simulink model "gm_sampleModel1831_sub"  (R2023a)
settings: Solver=VariableStepAuto  StartTime=0.0  StopTime=10.0  RelTol=1e-3
libraries: simulink x1
settings Model: Creator=user1  LastModifiedBy=user1
settings OptimizationCC: BlockReduction=off  ConditionallyExecuteInputs=off
settings DebuggingCC: InheritedTsInSrcMsg=none

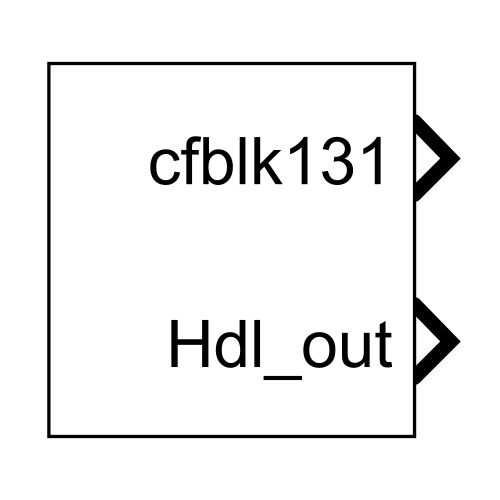
[thumbnail: Simulink's stored preview of the top-level diagram]
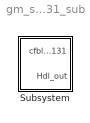
== system gm_sampleModel1831_sub ==
  Subsystem : Subsystem

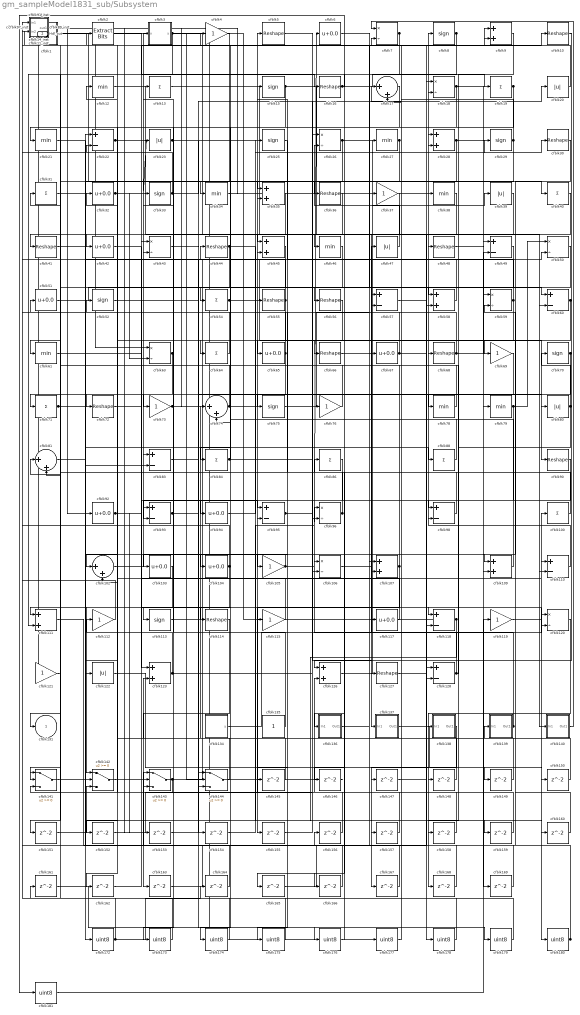
== system gm_sampleModel1831_sub/Subsystem ==
  cfblk1 : Subsystem  mask(Detect Rise Nonnegative){vinit=double(0), InputProcessing=Elements as channels (sample based), OutDataTypeStr=uint8}
      mask prompts: vinit "Simulink:masks:InitialCondition_MP"; InputProcessing "Simulink:masks:InputProcessing_MP"; OutDataTypeStr "Simulink:masks:OutputDataType_MP"
      mask help: Simulink:masks:DetectRiseNonnegative_MD
      mask init:
      | InputProcessing = 'Elements as channels (sample based)';
      | OutDataTypeStr = 'uint8';
      | vinit = double(0);
      mask TypeOptions InputProcessing: Simulink:masks:ColumnsAsChannelsFrameBased | Simulink:masks:ElementsAsChannelsSampleBased
      mask TypeOptions OutDataTypeStr: Simulink:masks:uint8 | Simulink:masks:boolean
      mask Display: fprintf('U >= 0\n&  NOT\nU/z >= 0')
  cfblk{5,10,16,30,36,41,44,48,55..56,66,68,72,90,114,127} (16 alike) : Reshape
  cfblk{13,19,31,40,54,64,71,84,86,88,100} (11 alike) : Sum  Inputs=+  OutDataTypeStr=uint8
  cfblk{17,74,81,102} (4 alike) : Sum  Inputs=|++  OutDataTypeStr=uint8
  cfblk{6,32,42,51,65,67,92,94,103..104,117} (11 alike) : Bias  Bias=0.0  SaturateOnIntegerOverflow=off
  cfblk{4,37,69,73,76,105,112,115,119,121} (10 alike) : Gain  OutDataTypeStr=uint8
  cfblk{7,18,26,43,50,59,63,96,106,120} (10 alike) : Product  Inputs=*/  OutDataTypeStr=uint8  RndMeth=Zero  SaturateOnIntegerOverflow=on
  cfblk{9,28,35,45,58,107,109,111,123,126} (10 alike) : Sum  OutDataTypeStr=uint8
  cfblk108_inst : Subsystem
  cfblk{22,49,57,60,83,93,95,98,110,118,128} (11 alike) : Sum  Inputs=+-  OutDataTypeStr=uint8
  cfblk{8,15,25,29,33,52,70,75,113} (9 alike) : Signum
  cfblk116_inst : Subsystem
  cfblk11_inst : Subsystem
  cfblk{12,21,27,34,38,46,61,78..79} (9 alike) : MinMax  OutDataTypeStr=uint8
  cfblk{20,23,39,47,80,122} (6 alike) : Abs  OutDataTypeStr=uint8  SaturateOnIntegerOverflow=off
  cfblk134 : Subsystem  mask(Counter Free-Running){NumBits=double(16), tsamp=double(-1)}
      mask prompts: NumBits "Simulink:masks:NumberOfBits_MP"; tsamp "Simulink:masks:SampleTime_MP"
      mask help: Simulink:masks:CounterFreeRunning_MD
  cfblk135 : Constant  OutDataTypeStr=uint8  SampleTime=-1
  cfblk136 : Subsystem
  cfblk137 : Subsystem
  cfblk138 : Subsystem
  cfblk139 : Subsystem
  cfblk140 : Subsystem
  cfblk{141..144} (4 alike) : Switch  OutDataTypeStr=uint8  SaturateOnIntegerOverflow=off  InputSameDT=off
  cfblk{145..169} (25 alike) : Delay  SampleTime=1
  cfblk14_inst : Subsystem
  cfblk{172..181} (10 alike) : DataTypeConversion  OutDataTypeStr=uint8  SaturateOnIntegerOverflow=off  RndMeth=Floor
  cfblk2 : simulink/Logic and Bit Operations/Extract Bits  bitsToExtract=Upper half  numBits=8  bitIdxRange=[0 7]  outScalingMode=Preserve fixed-point scaling
      settings: LibrarySourceBlock=|
      | hdlsllib/Logic and Bit
      | Operations/Extract Bits
  cfblk3 : Subsystem  mask(Compare To Zero){relop=<=, OutDataTypeStr=uint8, ZeroCross=on}
      mask prompts: relop "Simulink:masks:Operator_MP"; OutDataTypeStr "Simulink:masks:OutputDataType_MP"; ZeroCross "Simulink:masks:EnableZerocrossingDetection_MP"
      mask help: Simulink:masks:CompareToZero_MD
      mask init:
      | OutDataTypeStr = 'uint8';
      | ZeroCross = 'on';
      | blkName = 'sampleModel1831_sub/Subsystem/cfblk3';
      | relop = '<=';
      | setValue = 'fixdt(0, 8)';
      mask TypeOptions relop: == | ~= | < | <= | >= | >
      mask TypeOptions OutDataTypeStr: Simulink:masks:uint8 | Simulink:masks:boolean
      mask Callback ZeroCross: sl('zeroCrossEnable', gcbh);
      mask Display: disp([relop,' 0'])
  cfblk89_inst : Subsystem
  cfblk91_inst : Subsystem
  cfblk97_inst : Subsystem
  cfblk131 : Outport  OutDataTypeStr=uint8  SampleTime=1  VectorParamsAs1DForOutWhenUnconnected=off
  Hdl_out : Outport  Port=2  OutDataTypeStr=uint8  SampleTime=1
  wires:
  cfblk1/1(Y) -> cfblk40/1
  cfblk10/1 -> cfblk126/1
  cfblk100/1 -> cfblk108_inst/2(in2)
  cfblk102/1 -> cfblk3/1(u)
  cfblk103/1 -> cfblk142/1
  cfblk104/1 -> cfblk97_inst/2(in2), cfblk111/1
  cfblk105/1 -> cfblk6/1, cfblk103/1
  cfblk106/1 -> cfblk39/1
  cfblk107/1 -> cfblk43/2, cfblk155/1
  cfblk108_inst/1(out1) -> cfblk121/1
  cfblk109/1 -> cfblk44/1
  cfblk11_inst/1(out1) -> cfblk154/1
  cfblk110/1 -> cfblk8/1
  cfblk111/1 -> cfblk156/1
  cfblk112/1 -> cfblk116_inst/2(in2)
  cfblk113/1 -> cfblk118/1
  cfblk114/1 -> cfblk163/1
  cfblk115/1 -> cfblk116_inst/1(in1)
  cfblk116_inst/1(out1) -> cfblk63/1
  cfblk117/1 -> cfblk32/1
  cfblk118/1 -> cfblk165/1, Hdl_out/1
  cfblk119/1 -> cfblk180/1
  cfblk12/1 -> cfblk137/1(In1)
  cfblk120/1 -> cfblk168/1
  cfblk121/1 -> cfblk31/1
  cfblk122/1 -> cfblk148/1
  cfblk123/1 -> cfblk28/1, cfblk112/1
  cfblk126/1 -> cfblk29/1
  cfblk127/1 -> cfblk18/1
  cfblk128/1 -> cfblk68/1, cfblk47/1
  cfblk13/1 -> cfblk46/1
  cfblk134/1(y) -> cfblk100/1
  cfblk135/1 -> cfblk83/1
  cfblk136/1(Out1) -> cfblk67/1
  cfblk137/1(Out1) -> cfblk149/1
  cfblk138/1(Out1) -> cfblk167/1
  cfblk139/1(Out1) -> cfblk98/2, cfblk106/1
  cfblk14_inst/1(out1) -> cfblk92/1
  cfblk140/1(Out1) -> cfblk7/1
  cfblk141/1 -> cfblk50/2
  cfblk142/1 -> cfblk143/1
  cfblk143/1 -> cfblk5/1, cfblk141/3
  cfblk144/1 -> cfblk123/2
  cfblk145/1 -> cfblk22/2
  cfblk146/1 -> cfblk1/1(U)
  cfblk147/1 -> cfblk9/1
  cfblk148/1 -> cfblk35/2
  cfblk149/1 -> cfblk7/2
  cfblk15/1 -> cfblk140/1(In1), cfblk54/1
  cfblk150/1 -> cfblk74/1
  cfblk151/1 -> cfblk142/3
  cfblk152/1 -> cfblk26/1
  cfblk153/1 -> cfblk45/2
  cfblk154/1 -> cfblk96/1
  cfblk155/1 -> cfblk110/1
  cfblk156/1 -> cfblk143/2
  cfblk157/1 -> cfblk126/2
  cfblk158/1 -> cfblk102/2
  cfblk159/1 -> cfblk95/2
  cfblk16/1 -> cfblk181/1, cfblk19/1
  cfblk160/1 -> cfblk59/2
  cfblk161/1 -> cfblk179/1
  cfblk162/1 -> cfblk107/2
  cfblk163/1 -> cfblk58/2
  cfblk164/1 -> cfblk43/1
  cfblk165/1 -> cfblk128/2
  cfblk166/1 -> cfblk143/3
  cfblk167/1 -> cfblk142/2
  cfblk168/1 -> cfblk57/1
  cfblk169/1 -> cfblk91_inst/2(in2)
  cfblk17/1 -> cfblk162/1
  cfblk172/1 -> cfblk108_inst/1(in1), cfblk164/1
  cfblk173/1 -> cfblk81/1
  cfblk174/1 -> cfblk81/2
  cfblk175/1 -> cfblk161/1
  cfblk176/1 -> cfblk86/1
  cfblk177/1 -> cfblk57/2
  cfblk178/1 -> cfblk89_inst/1(in1)
  cfblk179/1 -> cfblk89_inst/2(in2)
  cfblk18/1 -> cfblk49/1, cfblk158/1, cfblk21/1
  cfblk180/1 -> cfblk107/1, cfblk139/1(In1)
  cfblk181/1 -> cfblk119/1
  cfblk19/1 -> cfblk42/1, cfblk173/1
  cfblk2/1 -> cfblk16/1
  cfblk20/1 -> cfblk2/1
  cfblk21/1 -> cfblk157/1
  cfblk22/1 -> cfblk35/1, cfblk169/1
  cfblk23/1 -> cfblk144/1, cfblk59/1
  cfblk25/1 -> cfblk65/1
  cfblk26/1 -> cfblk28/2, cfblk84/1
  cfblk27/1 -> cfblk93/2, cfblk45/1
  cfblk28/1 -> cfblk151/1, cfblk150/1
  cfblk29/1 -> cfblk97_inst/1(in1), cfblk61/1
  cfblk3/1(y) -> cfblk178/1, cfblk141/2
  cfblk30/1 -> cfblk109/1
  cfblk31/1 -> cfblk34/1
  cfblk32/1 -> cfblk23/1, cfblk63/2, cfblk106/2
  cfblk33/1 -> cfblk14_inst/1(in1), cfblk18/2
  cfblk34/1 -> cfblk25/1
  cfblk35/1 -> cfblk72/1
  cfblk36/1 -> cfblk96/2
  cfblk37/1 -> cfblk146/1
  cfblk38/1 -> cfblk41/1
  cfblk39/1 -> cfblk98/1
  cfblk4/1 -> cfblk73/1
  cfblk40/1 -> cfblk105/1
  cfblk41/1 -> cfblk83/2
  cfblk42/1 -> cfblk118/2
  cfblk43/1 -> cfblk78/1
  cfblk44/1 -> cfblk144/3, cfblk160/1, cfblk159/1
  cfblk45/1 -> cfblk74/2
  cfblk46/1 -> cfblk94/1
  cfblk47/1 -> cfblk26/2
  cfblk48/1 -> cfblk79/1
  cfblk49/1 -> cfblk71/1
  cfblk5/1 -> cfblk69/1
  cfblk50/1 -> cfblk131/1
  cfblk51/1 -> cfblk60/1
  cfblk52/1 -> cfblk117/1
  cfblk54/1 -> cfblk90/1, cfblk37/1
  cfblk55/1 -> cfblk14_inst/2(in2), cfblk64/1
  cfblk56/1 -> cfblk102/1
  cfblk57/1 -> cfblk128/1
  cfblk58/1 -> cfblk15/1
  cfblk59/1 -> cfblk48/1, cfblk144/2
  cfblk6/1 -> cfblk60/2
  cfblk60/1 -> cfblk174/1, cfblk104/1
  cfblk61/1 -> cfblk95/1
  cfblk63/1 -> cfblk141/1, cfblk152/1
  cfblk64/1 -> cfblk12/1
  cfblk65/1 -> cfblk52/1, cfblk114/1
  cfblk66/1 -> cfblk10/1
  cfblk67/1 -> cfblk91_inst/1(in1), cfblk120/2
  cfblk68/1 -> cfblk49/2, cfblk17/1
  cfblk69/1 -> cfblk136/1(In1)
  cfblk7/1 -> cfblk56/1, cfblk111/2
  cfblk70/1 -> cfblk122/1, cfblk110/2
  cfblk71/1 -> cfblk109/2, cfblk88/1
  cfblk72/1 -> cfblk9/2
  cfblk73/1 -> cfblk75/1, cfblk113/1
  cfblk74/1 -> cfblk80/1, cfblk147/1, cfblk13/1
  cfblk75/1 -> cfblk27/1
  cfblk76/1 -> cfblk22/1
  cfblk78/1 -> cfblk51/1
  cfblk79/1 -> cfblk93/1, cfblk50/1
  cfblk8/1 -> cfblk66/1, cfblk36/1, cfblk166/1
  cfblk80/1 -> cfblk70/1, cfblk138/1(In1)
  cfblk81/1 -> cfblk172/1
  cfblk83/1 -> cfblk115/1
  cfblk84/1 -> cfblk4/1, cfblk120/1
  cfblk86/1 -> cfblk175/1
  cfblk88/1 -> cfblk11_inst/1(in1)
  cfblk89_inst/1(out1) -> cfblk177/1
  cfblk9/1 -> cfblk58/1
  cfblk90/1 -> cfblk145/1
  cfblk91_inst/1(out1) -> cfblk76/1
  cfblk92/1 -> cfblk123/1, cfblk153/1
  cfblk93/1 -> cfblk33/1, cfblk176/1
  cfblk94/1 -> cfblk30/1
  cfblk95/1 -> cfblk20/1, cfblk127/1
  cfblk96/1 -> cfblk55/1, cfblk11_inst/2(in2)
  cfblk97_inst/1(out1) -> cfblk38/1
  cfblk98/1 -> cfblk17/2

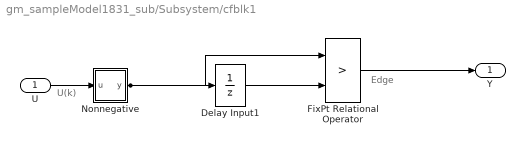
== system gm_sampleModel1831_sub/Subsystem/cfblk1 ==
  note: U(k)
  note: Edge
  U : Inport  OutDataTypeStr=uint8  SampleTime=1
  Delay Input1 : UnitDelay  Description=Store in Global RAM  DisableCoverage=on  InitialCondition=vinit  SampleTime=-1  HasFrameUpgradeWarning=on
  FixPt Relational Operator : RelationalOperator  Operator=>  OutDataTypeStr=fixdt(0, 8)  ZeroCross=off  InputSameDT=off
  Nonnegative : Subsystem  mask(Compare To Zero){relop=>=, OutDataTypeStr=boolean, ZeroCross=off}
      mask prompts: relop "Simulink:masks:Operator_MP"; OutDataTypeStr "Simulink:masks:OutputDataType_MP"; ZeroCross "Simulink:masks:EnableZerocrossingDetection_MP"
      mask help: Simulink:masks:CompareToZero_MD
      mask init:
      | OutDataTypeStr = 'boolean';
      | ZeroCross = 'off';
      | blkName = 'sampleModel1831_sub/Subsystem/cfblk1/Nonnegative';
      | relop = '>=';
      | setValue = 'boolean';
      mask TypeOptions relop: == | ~= | < | <= | >= | >
      mask TypeOptions OutDataTypeStr: Simulink:masks:uint8 | Simulink:masks:boolean
      mask Callback ZeroCross: sl('zeroCrossEnable', gcbh);
      mask Display: disp([relop,' 0'])
  Y : Outport  SampleTime=1
  wires:
  U/1 -> Nonnegative/1(u)
  Delay Input1/1 -> FixPt Relational Operator/2
  FixPt Relational Operator/1 -> Y/1
  Nonnegative/1(y) -> FixPt Relational Operator/1, Delay Input1/1

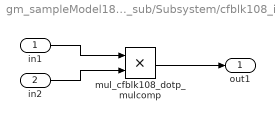
== system gm_sampleModel1831_sub/Subsystem/cfblk108_inst ==
  in1 : Inport  OutDataTypeStr=uint8  SampleTime=1
  in2 : Inport  Port=2  OutDataTypeStr=uint8  SampleTime=1
  mul_cfblk108_dotp_mulcomp : Product  Inputs=**  OutDataTypeStr=uint8  SampleTime=1
  out1 : Outport  OutDataTypeStr=uint8  SampleTime=1
  wires:
  in1/1 -> mul_cfblk108_dotp_mulcomp/1
  in2/1 -> mul_cfblk108_dotp_mulcomp/2
  mul_cfblk108_dotp_mulcomp/1 -> out1/1

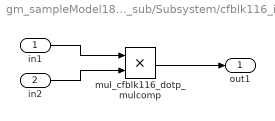
== system gm_sampleModel1831_sub/Subsystem/cfblk116_inst ==
  in1 : Inport  OutDataTypeStr=uint8  SampleTime=1
  in2 : Inport  Port=2  OutDataTypeStr=uint8  SampleTime=1
  mul_cfblk116_dotp_mulcomp : Product  Inputs=**  OutDataTypeStr=uint8  SampleTime=1
  out1 : Outport  OutDataTypeStr=uint8  SampleTime=1
  wires:
  in1/1 -> mul_cfblk116_dotp_mulcomp/1
  in2/1 -> mul_cfblk116_dotp_mulcomp/2
  mul_cfblk116_dotp_mulcomp/1 -> out1/1

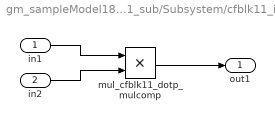
== system gm_sampleModel1831_sub/Subsystem/cfblk11_inst ==
  in1 : Inport  OutDataTypeStr=uint8  SampleTime=1
  in2 : Inport  Port=2  OutDataTypeStr=uint8  SampleTime=1
  mul_cfblk11_dotp_mulcomp : Product  Inputs=**  OutDataTypeStr=uint8  SampleTime=1
  out1 : Outport  OutDataTypeStr=uint8  SampleTime=1
  wires:
  in1/1 -> mul_cfblk11_dotp_mulcomp/1
  in2/1 -> mul_cfblk11_dotp_mulcomp/2
  mul_cfblk11_dotp_mulcomp/1 -> out1/1

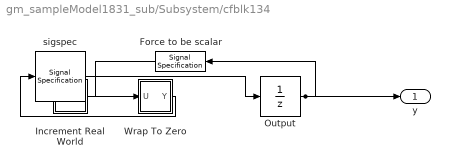
== system gm_sampleModel1831_sub/Subsystem/cfblk134 ==
  Force to be scalar : SignalSpecification  DisableCoverage=on  Dimensions=1
  Increment Real World : Subsystem  mask(Real World Value Increment){}
      mask help: Simulink:masks:RealWorldValueIncrement_MD
      mask Display: disp('V++')
  Output : UnitDelay  InitialCondition=0.0  SampleTime=tsamp  HasFrameUpgradeWarning=on
  Wrap To Zero : Subsystem  mask(Wrap To Zero){Threshold=double(65535)}
      mask prompts: Threshold "Simulink:masks:Threshold_MP"
      mask help: Simulink:masks:WrapToZero_MD
  sigspec : SignalSpecification  OutDataTypeStr=uint16  Dimensions=1
  y : Outport  SampleTime=1
  wires:
  Force to be scalar/1 -> Increment Real World/1(u)
  Increment Real World/1(y) -> Wrap To Zero/1(U)
  Output/1 -> Force to be scalar/1, y/1
  Wrap To Zero/1(Y) -> sigspec/1
  sigspec/1 -> Output/1

== system gm_sampleModel1831_sub/Subsystem/cfblk136 ==
  In1 : Inport  OutDataTypeStr=uint8  PortDimensions=1  SampleTime=1
  Out1 : Outport  SampleTime=1
  wires:
  In1/1 -> Out1/1

== system gm_sampleModel1831_sub/Subsystem/cfblk137 ==
  In1 : Inport  OutDataTypeStr=uint8  PortDimensions=1  SampleTime=1
  Out1 : Outport  SampleTime=1
  wires:
  In1/1 -> Out1/1

== system gm_sampleModel1831_sub/Subsystem/cfblk138 ==
  In1 : Inport  OutDataTypeStr=uint8  PortDimensions=1  SampleTime=1
  Out1 : Outport  SampleTime=1
  wires:
  In1/1 -> Out1/1

== system gm_sampleModel1831_sub/Subsystem/cfblk139 ==
  In1 : Inport  OutDataTypeStr=uint8  PortDimensions=1  SampleTime=1
  Out1 : Outport  SampleTime=1
  wires:
  In1/1 -> Out1/1

== system gm_sampleModel1831_sub/Subsystem/cfblk140 ==
  In1 : Inport  OutDataTypeStr=uint8  PortDimensions=1  SampleTime=1
  Out1 : Outport  SampleTime=1
  wires:
  In1/1 -> Out1/1

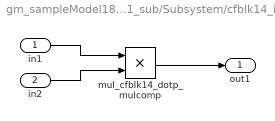
== system gm_sampleModel1831_sub/Subsystem/cfblk14_inst ==
  in1 : Inport  OutDataTypeStr=uint8  SampleTime=1
  in2 : Inport  Port=2  OutDataTypeStr=uint8  SampleTime=1
  mul_cfblk14_dotp_mulcomp : Product  Inputs=**  OutDataTypeStr=uint8  SampleTime=1
  out1 : Outport  OutDataTypeStr=uint8  SampleTime=1
  wires:
  in1/1 -> mul_cfblk14_dotp_mulcomp/1
  in2/1 -> mul_cfblk14_dotp_mulcomp/2
  mul_cfblk14_dotp_mulcomp/1 -> out1/1

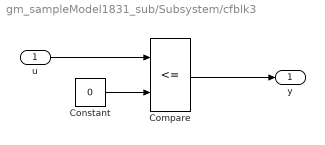
== system gm_sampleModel1831_sub/Subsystem/cfblk3 ==
  u : Inport  OutDataTypeStr=uint8  SampleTime=1
  Compare : RelationalOperator  Operator=<=  OutDataTypeStr=fixdt(0, 8)
  Constant : Constant  DisableCoverage=on  Value=0  OutDataTypeStr=Inherit: Inherit via back propagation  SampleTime=-1  PreserveConstantTs=on
  y : Outport  SampleTime=1
  wires:
  u/1 -> Compare/1
  Compare/1 -> y/1
  Constant/1 -> Compare/2

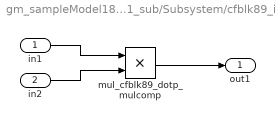
== system gm_sampleModel1831_sub/Subsystem/cfblk89_inst ==
  in1 : Inport  OutDataTypeStr=uint8  SampleTime=1
  in2 : Inport  Port=2  OutDataTypeStr=uint8  SampleTime=1
  mul_cfblk89_dotp_mulcomp : Product  Inputs=**  OutDataTypeStr=uint8  SampleTime=1
  out1 : Outport  OutDataTypeStr=uint8  SampleTime=1
  wires:
  in1/1 -> mul_cfblk89_dotp_mulcomp/1
  in2/1 -> mul_cfblk89_dotp_mulcomp/2
  mul_cfblk89_dotp_mulcomp/1 -> out1/1

== system gm_sampleModel1831_sub/Subsystem/cfblk91_inst ==
  in1 : Inport  OutDataTypeStr=uint8  SampleTime=1
  in2 : Inport  Port=2  OutDataTypeStr=uint8  SampleTime=1
  mul_cfblk91_dotp_mulcomp : Product  Inputs=**  OutDataTypeStr=uint8  SampleTime=1
  out1 : Outport  OutDataTypeStr=uint8  SampleTime=1
  wires:
  in1/1 -> mul_cfblk91_dotp_mulcomp/1
  in2/1 -> mul_cfblk91_dotp_mulcomp/2
  mul_cfblk91_dotp_mulcomp/1 -> out1/1

== system gm_sampleModel1831_sub/Subsystem/cfblk97_inst ==
  in1 : Inport  OutDataTypeStr=uint8  SampleTime=1
  in2 : Inport  Port=2  OutDataTypeStr=uint8  SampleTime=1
  mul_cfblk97_dotp_mulcomp : Product  Inputs=**  OutDataTypeStr=uint8  SampleTime=1
  out1 : Outport  OutDataTypeStr=uint8  SampleTime=1
  wires:
  in1/1 -> mul_cfblk97_dotp_mulcomp/1
  in2/1 -> mul_cfblk97_dotp_mulcomp/2
  mul_cfblk97_dotp_mulcomp/1 -> out1/1

== system gm_sampleModel1831_sub/Subsystem/cfblk1/Nonnegative ==
  u : Inport  OutDataTypeStr=uint8  SampleTime=1
  Compare : RelationalOperator  OutDataTypeStr=boolean  ZeroCross=off
  Constant : Constant  DisableCoverage=on  Value=0  OutDataTypeStr=Inherit: Inherit via back propagation  SampleTime=-1  PreserveConstantTs=on
  y : Outport  SampleTime=1
  wires:
  u/1 -> Compare/1
  Compare/1 -> y/1
  Constant/1 -> Compare/2

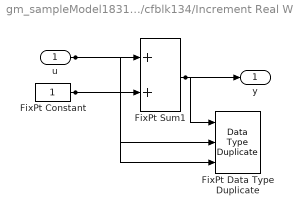
== system gm_sampleModel1831_sub/Subsystem/cfblk134/Increment Real World ==
  u : Inport  OutDataTypeStr=uint16  SampleTime=1
  FixPt Constant : Constant  DisableCoverage=on  OutDataTypeStr=Inherit: Inherit via back propagation  SampleTime=-1
  FixPt Data Type Duplicate : DataTypeDuplicate  DisableCoverage=on  NumInputPorts=3
  FixPt Sum1 : Sum  InputSameDT=on  OutDataTypeStr=Inherit: Inherit via back propagation  LockScale=on
  y : Outport  SampleTime=1
  wires:
  u/1 -> FixPt Sum1/1, FixPt Data Type Duplicate/2
  FixPt Constant/1 -> FixPt Sum1/2, FixPt Data Type Duplicate/3
  FixPt Sum1/1 -> FixPt Data Type Duplicate/1, y/1

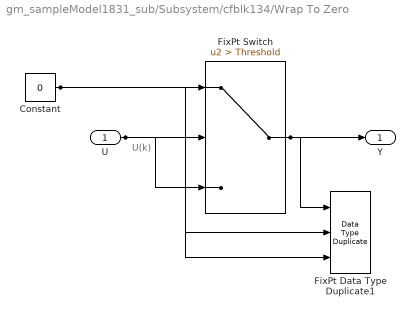
== system gm_sampleModel1831_sub/Subsystem/cfblk134/Wrap To Zero ==
  note: U(k)
  U : Inport  OutDataTypeStr=uint16  SampleTime=1
  Constant : Constant  DisableCoverage=on  Value=0  OutDataTypeStr=Inherit: Inherit via back propagation  SampleTime=-1
  FixPt Data Type Duplicate1 : DataTypeDuplicate  DisableCoverage=on  NumInputPorts=3
  FixPt Switch : Switch  Criteria=u2 > Threshold  Threshold=Threshold  OutDataTypeStr=Inherit: Inherit via back propagation  ZeroCross=off  SaturateOnIntegerOverflow=off  InputSameDT=off
  Y : Outport  SampleTime=1
  wires:
  U/1 -> FixPt Switch/3, FixPt Switch/2, FixPt Data Type Duplicate1/2
  Constant/1 -> FixPt Switch/1, FixPt Data Type Duplicate1/3
  FixPt Switch/1 -> FixPt Data Type Duplicate1/1, Y/1
